simulink model "semi_controlled_bridge_rectifier"  (R2022a)
settings: Solver=VariableStepAuto  StartTime=0.0  StopTime=0.1  RelTol=1e-3
libraries: spsVoltageMeasurementLib x4, spsCurrentMeasurementLib x2, spsDiodeLib x2, spsThyristorLib x2, spsACVoltageSourceLib x1, spsGroundLib x1, spsParallelRLCBranchLib x1, spspowerguiLib x1
settings Model: Creator=P.O.M.G  LastModifiedBy=P.O.M.G

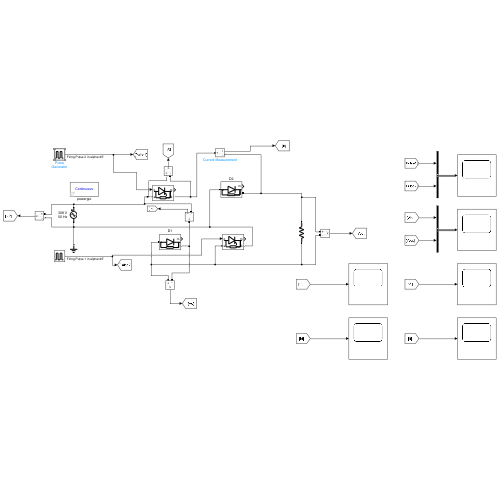
[thumbnail: Simulink's stored preview of the top-level diagram]
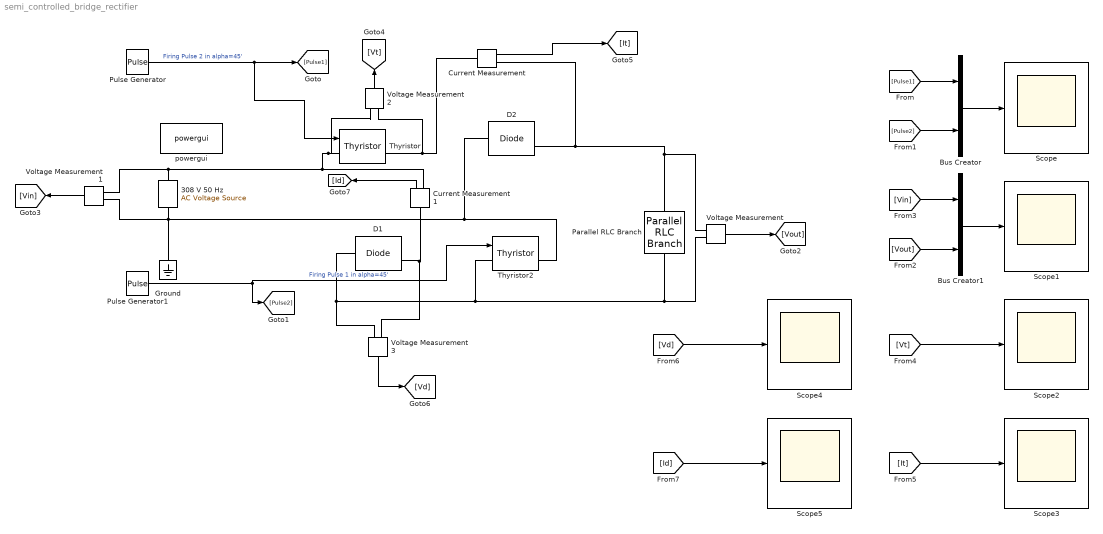
== system semi_controlled_bridge_rectifier ==
  308 V 50 Hz : spsACVoltageSourceLib/AC Voltage Source  Amplitude=308  Phase=0  Frequency=50  SampleTime=0  Measurements=None  BusType=swing  Pref=10e3  Qref=0  Qmin=-inf  Qmax=+inf
  Bus Creator : BusCreator  Inputs=2
  Bus Creator1 : BusCreator  Inputs=2
  Current Measurement : spsCurrentMeasurementLib/Current Measurement  PhasorSimulation=off  OutputType=Complex  PSBequivalent=0
  Current Measurement1 : spsCurrentMeasurementLib/Current Measurement  PhasorSimulation=off  OutputType=Complex  PSBequivalent=0
  D1 : spsDiodeLib/Diode  Ron=0.001  Lon=0  Vf=0.8  IC=0  UseSnubber=0  Rs=500  Cs=250e-9  Measurements=on
  D2 : spsDiodeLib/Diode  Ron=0.001  Lon=0  Vf=0.8  IC=0  UseSnubber=0  Rs=500  Cs=250e-9  Measurements=on
  Ground : spsGroundLib/Ground  LConnTagsString=a
  Parallel RLC Branch : spsParallelRLCBranchLib/Parallel RLC Branch  LConnTagsString=a  RConnTagsString=__new0  BranchType=R  Resistance=10  Inductance=1e-3  SetiL0=off  InitialCurrent=0  Capacitance=1e-6  Setx0=off  InitialVoltage=0  Measurements=None
  Pulse Generator : DiscretePulseGenerator  PulseType=Time based  Period=0.02  PulseWidth=5  PhaseDelay=.0025
  Pulse Generator1 : DiscretePulseGenerator  PulseType=Time based  Period=0.02  PulseWidth=5  PhaseDelay=0.05
  Scope{,1..5} (6 alike) : Scope
  Thyristor : spsThyristorLib/Thyristor  Ron=0.001  Lon=0  Vf=0.8  IC=0  Rs=500  Cs=250e-9  Measurements=on
  Thyristor2 : spsThyristorLib/Thyristor  Ron=0.001  Lon=0  Vf=0.8  IC=0  Rs=500  Cs=250e-9  Measurements=on
  Voltage Measurement{,1..3} (4 alike) : spsVoltageMeasurementLib/Voltage Measurement  PhasorSimulation=off  OutputType=Complex  PSBequivalent=0
  powergui : spspowerguiLib/powergui  Priority=1  SimulationMode=Continuous  SampleTime=50e-6  frequency=60  Iterations=50  frequencyindice=50  Pbase=100e6  ErrMax=1e-4  UnitsV=kV  UnitsW=MW  buscounter=0  FunctionMessages=off  echomessages=off  EnableUseOfTLC=off  CurrentSourceSwitches=off  DisableSnubberDevices=off  DisableRonSwitches=off  DisableVfSwitches=off  DisplayEquations=off  AutomaticDiscreteSolvers=off  SolverType=Tustin/Backward Euler (TBE)  Interpol=off  ExternalGateDelay=off  methode=off  Ts=100  x0status=blocks  SPID=on  SwTol=0  HookPort=off  NonlinearTolerance=1e-4  nMaxIteration=100  ContinueOnMaxIteration=off  RestoreLinks=warning  ResistiveCurrentMeasurement=off  Frange=[0:2:500]  Ylog=off  Xlog=on  ShowGrid=off  save=off  variable=ZData  structure=0  ZoomFFT=off  StartTime=0.0  cycles=1  DisplayStyle=1  fundamental=60  FreqAxis=off  MaxFrequency=1000  frequencyindicesteady=1  RmsSteady=1  display=off
  wires:
  Bus Creator1/1 -> Scope1/1
  [Vt] -> Scope2/1
  Voltage Measurement2/1 -> [Vt]
  [It] -> Scope3/1
  Voltage Measurement/1 -> [Vout]
  [Pulse2] -> Bus Creator/2
  [Vin] -> Bus Creator1/1
  [Pulse1] -> Bus Creator/1
  Current Measurement/1 -> [It]
  Bus Creator/1 -> Scope/1
  Pulse Generator/1 -> Thyristor/1, [Pulse1]  "Firing Pulse 2 in alpha=45'"
  Voltage Measurement1/1 -> [Vin]
  [Vout] -> Bus Creator1/2
  Pulse Generator1/1 -> Thyristor2/1, [Pulse2]  "Firing Pulse 1 in alpha=45'"
  [Vd] -> Scope4/1
  [Id] -> Scope5/1
  Voltage Measurement3/1 -> [Vd]
  Current Measurement1/1 -> [Id]
  connections:
  Parallel RLC Branch/LConn1 -- D2/RConn1 -- Current Measurement/RConn1 -- Voltage Measurement/LConn1
  Thyristor/LConn1 -- Current Measurement1/RConn1 -- 308 V 50 Hz/RConn1 -- Voltage Measurement1/LConn1 -- Voltage Measurement2/LConn1
  Current Measurement/LConn1 -- Voltage Measurement2/LConn2 -- Thyristor/RConn1
  Thyristor2/RConn1 -- D2/LConn1 -- Voltage Measurement1/LConn2 -- 308 V 50 Hz/LConn1 -- Ground/LConn1
  Voltage Measurement/LConn2 -- Parallel RLC Branch/RConn1 -- D1/LConn1 -- Voltage Measurement3/LConn1 -- Thyristor2/LConn1
  D1/RConn1 -- Current Measurement1/LConn1 -- Voltage Measurement3/LConn2
